simulink model "hw9_11_59_b"  (R2018b)
settings: Solver=FixedStepAuto  StartTime=0.0  StopTime=5  FixedStep=0.001  RelTol=1e-3
settings Model: Creator=HyperDrive  LastModifiedBy=HyperDrive

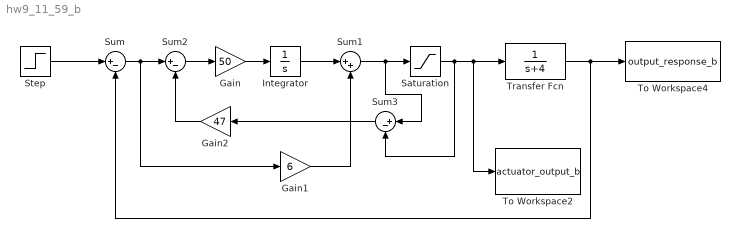
== system hw9_11_59_b ==
  Gain : Gain  Gain=50
  Gain1 : Gain  Gain=6
  Gain2 : Gain  Gain=47
  Integrator : Integrator
  Saturation : Saturate  UpperLimit=5  LowerLimit=-5
  Step : Step  Time=0  SampleTime=0
  Sum : Sum  Inputs=|+-
  Sum1 : Sum  Inputs=|++
  Sum2 : Sum  Inputs=|+-
  Sum3 : Sum  Inputs=|+-
  To Workspace2 : ToWorkspace  VariableName=actuator_output_b  SaveFormat=Structure With Time  SampleTime=-1
  To Workspace4 : ToWorkspace  VariableName=output_response_b  SaveFormat=Structure With Time  SampleTime=-1
  Transfer Fcn : TransferFcn  Denominator=[1 4]
  wires:
  Integrator/1 -> Sum1/1
  Gain/1 -> Integrator/1
  Step/1 -> Sum/1
  Sum1/1 -> Sum3/1, Saturation/1
  Sum/1 -> Sum2/1, Gain1/1
  Gain1/1 -> Sum1/2
  Saturation/1 -> To Workspace2/1, Transfer Fcn/1, Sum3/2
  Transfer Fcn/1 -> Sum/2, To Workspace4/1
  Sum2/1 -> Gain/1
  Sum3/1 -> Gain2/1
  Gain2/1 -> Sum2/2
